simulink model "Project3_Trial"  (R2023b)
settings: Solver=VariableStepAuto  StartTime=0.0  StopTime=100.0  MaxStep=0.01  RelTol=1e-3
settings Model: Creator=LL  LastModifiedBy=LL

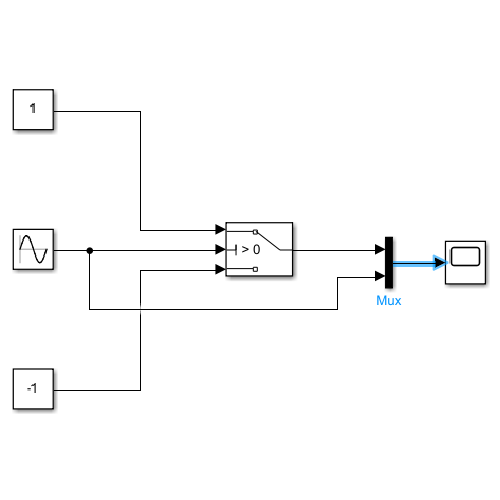
[thumbnail: Simulink's stored preview of the top-level diagram]
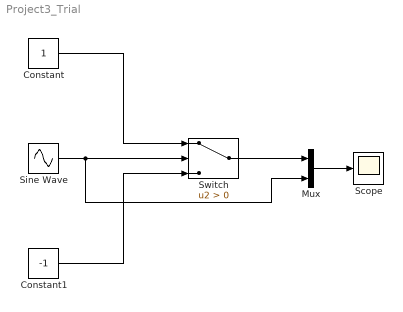
== system Project3_Trial ==
  Constant : Constant
  Constant1 : Constant  Value=-1
  Mux : Mux  Inputs=2
  Scope : Scope
  Sine Wave : Sin  SampleTime=0
  Switch : Switch  Criteria=u2 > Threshold  SaturateOnIntegerOverflow=off  InputSameDT=off
  wires:
  Sine Wave/1 -> Mux/2, Switch/2
  Constant/1 -> Switch/1
  Constant1/1 -> Switch/3
  Switch/1 -> Mux/1
  Mux/1 -> Scope/1
